simulink model "bench_test_racecar_shiftlight"  (R2023b)
settings: Solver=FixedStepDiscrete  StartTime=0.0  StopTime=inf  FixedStep=0.001  RelTol=1e-3  EnableMultiTasking=on
PreLoadFcn:
  | colow_ws2812
values from neighbouring files (symbols this model uses):
  all_off = [one_off one_off one_off one_off one_off one_off one_off one_off one_off one_off one_off one_off one_off one_off zeros]    [colow_ws2812.m]
  final_drive_ratio = 4.765    [colow_ws2812.m]
  red_day_all = [red_day red_day red_day red_day red_day red_day red_day red_day red_day red_day red_day red_day red_day red_day zeros]    [colow_ws2812.m]
  red_night_all = [red_night red_night red_night red_night red_night red_night red_night red_night red_night red_night red_night red_night red_night red_night zeros]    [colow_ws2812.m]
  stage1_day = [green_day linspace(20,20,288) green_day zeros]    [colow_ws2812.m]
  stage1_night = [green_night linspace(20,20,288) green_night zeros]    [colow_ws2812.m]
  stage2_day = [green_day green_day linspace(20,20,240) green_day green_day zeros]    [colow_ws2812.m]
  stage2_night = [green_night green_night linspace(20,20,240) green_night green_night zeros]    [colow_ws2812.m]
  stage3_day = [green_day green_day red_day linspace(20,20,192) red_day green_day green_day zeros]    [colow_ws2812.m]
  stage3_night = [green_night green_night red_night linspace(20,20,192) red_night green_night green_night zeros]    [colow_ws2812.m]
  stage4_day = [green_day green_day red_day red_day linspace(20,20,144) red_day red_day green_day green_day zeros]    [colow_ws2812.m]
  stage4_night = [green_night green_night red_night red_night linspace(20,20,144) red_night red_night green_night green_night zeros]    [colow_ws2812.m]
  stage5_day = [green_day green_day red_day red_day blue_day linspace(20,20,96) blue_day red_day red_day green_day green_day zeros]    [colow_ws2812.m]
  stage5_night = [green_night green_night red_night red_night blue_night linspace(20,20,96) blue_night red_night red_night green_night green_night zeros]    [colow_ws2812.m]
  stage6_day = [green_day green_day red_day red_day blue_day blue_day linspace(20,20,48) blue_day blue_day red_day red_day green_day green_day zeros]    [colow_ws2812.m]
  stage6_night = [green_night green_night red_night red_night blue_night blue_night linspace(20,20,48) blue_night blue_night red_night red_night green_night green_night zeros]    [colow_ws2812.m]
  stage7_day = [green_day green_day red_day red_day blue_day blue_day blue_day blue_day blue_day blue_day red_day red_day green_day green_day zeros]    [colow_ws2812.m]
  stage7_night = [green_night green_night red_night red_night blue_night blue_night blue_night blue_night blue_night blue_night red_night red_night green_night green_night zeros]    [colow_ws2812.m]
  tire_radius = 0.31265    [colow_ws2812.m]
undefined symbols (not defined in the file or in its folder): Down, epwmFrequency, GPTRIP1SEL, GPTRIP2SEL, TZ1, TZ2, Up
libraries: simulink x18, c2837xDlib x7, c280xlib x4, canmsglib x4, c2802xlib x1
settings Model: ExtModeTrigDuration=8  Creator=LinF  LastModifiedBy=LinF
settings OptimizationCC: DefaultUnderspecifiedDataType=single  EnhancedBackFolding=on  PassReuseOutputArgsAs=Individual arguments  MaxStackSize=1024  OptimizeBlockOrder=speed  DifferentSizesBufferReuse=on  OptimizationCustomize=off  EfficientTunableParamExpr=on
settings DebuggingCC: ParameterTunabilityLossMsg=error
settings HardwareCC: ProdBitPerChar=16  ProdBitPerInt=16  ProdBitPerPointer=32  ProdBitPerSizeT=32  ProdBitPerPtrDiffT=32  ProdLargestAtomicInteger=Integer  ProdLargestAtomicFloat=None  ProdWordSize=16  ProdLongLongMode=on  ProdHWDeviceType=Texas Instruments->C2000  HardwareBoardFeatureSet=SoCBlockset
settings ModelReferenceCC: ModelReferenceNumInstancesAllowed=Single
settings SFSimCC: MATLABDynamicMemAlloc=off
settings RTWCC: Description=Embedded Coder  SystemTargetFile=ert.tlc  HardwareBoard=TI Delfino F28379D LaunchPad  TemplateMakefile=ert_default_tmf  Toolchain=Texas Instruments Code Composer Studio (C2000)  CodeProfilingSaveOptions=MetricsOnly
settings CodeAppCC: ForceParamTrailComments=on  IgnoreCustomStorageClasses=off  OperatorAnnotations=on  SimulinkDataObjDesc=on  SFDataObjDesc=on  InsertBlockDesc=on
settings ERTTargetCC: CodeReplacementLibrary=TI C28x  ExtModeTransport=4  ExtModeStaticAlloc=on  ExtModeAutomaticAllocSize=off  ExtModeStaticAllocSize=10000  ExtModeMexFile=ext_xcp  ExtModeIntrfLevel=Level2 - Open

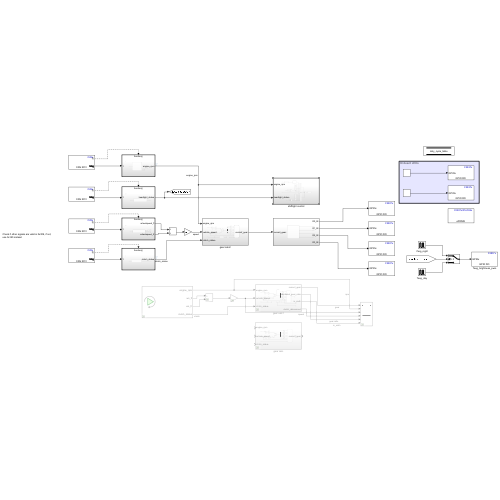
[thumbnail: Simulink's stored preview of the top-level diagram]
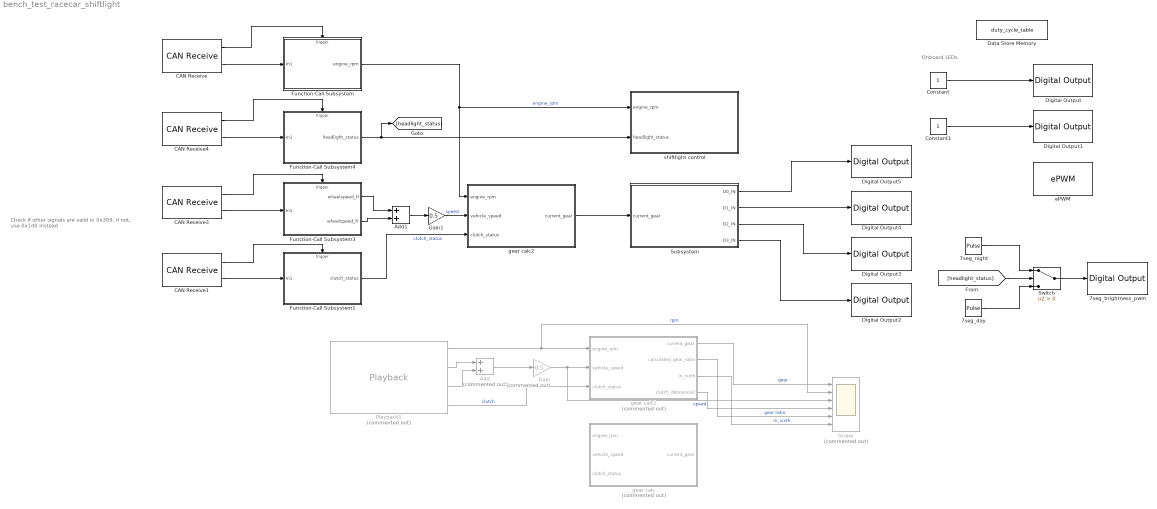
== system bench_test_racecar_shiftlight ==
  note: Check if other signals are valid in 0x309, if not,
      | use 0x1d0 instead
  note: Onboard LEDs
  7seg_brightness_pwm : c2837xDlib/Digital Output  GPIO_Number=GPIO128~GPIO135  GPIO_Bit0=off  GPIO_BIT0_Toggle=off  GPIO_Bit1=off  GPIO_BIT1_Toggle=off  GPIO_Bit2=on  GPIO_BIT2_Toggle=off  GPIO_Bit3=off  GPIO_BIT3_Toggle=off  GPIO_Bit4=off  GPIO_BIT4_Toggle=off  GPIO_Bit5=off  GPIO_BIT5_Toggle=off  GPIO_Bit6=off  GPIO_BIT6_Toggle=off  GPIO_Bit7=off  GPIO_BIT7_Toggle=off
  7seg_day : DiscretePulseGenerator  PulseType=Time based  Period=0.01  PulseWidth=40
  7seg_night : DiscretePulseGenerator  PulseType=Time based  Period=0.01  PulseWidth=90
  Add : Sum  Commented=on
  Add1 : Sum
  CAN Receive : c280xlib/CAN Receive  chipFamily=C280x  useModule=CAN_B  mailboxNo=0  messageID=hex2dec('17c')  messageType=Standard (11-bit identifier)  enableAcceptanceFiltering=off  messageIDMask=0  sampleTime=-1  dataType=CAN_MESSAGE_TYPE  outputAction=Output last received values  initValue=0  outputMessageID=off  outputMessageLength=off  outputMessageTimeStamp=off  postInterrupt=off  interruptLine=0
      settings: LibrarySourceBlock=c2837xDlib/CAN Receive
  CAN Receive1 : c280xlib/CAN Receive  chipFamily=C280x  useModule=CAN_B  mailboxNo=2  messageID=hex2dec('13c')  messageType=Standard (11-bit identifier)  enableAcceptanceFiltering=off  messageIDMask=0  sampleTime=-1  dataType=CAN_MESSAGE_TYPE  outputAction=Output last received values  initValue=0  outputMessageID=off  outputMessageLength=off  outputMessageTimeStamp=off  postInterrupt=off  interruptLine=0
      settings: LibrarySourceBlock=c2837xDlib/CAN Receive
  CAN Receive3 : c280xlib/CAN Receive  chipFamily=C280x  useModule=CAN_B  mailboxNo=3  messageID=hex2dec('1d0')  messageType=Standard (11-bit identifier)  enableAcceptanceFiltering=off  messageIDMask=0  sampleTime=-1  dataType=CAN_MESSAGE_TYPE  outputAction=Output last received values  initValue=0  outputMessageID=off  outputMessageLength=off  outputMessageTimeStamp=off  postInterrupt=off  interruptLine=0
      settings: LibrarySourceBlock=c2837xDlib/CAN Receive
  CAN Receive4 : c280xlib/CAN Receive  chipFamily=C280x  useModule=CAN_B  mailboxNo=4  messageID=hex2dec('164')  messageType=Standard (11-bit identifier)  enableAcceptanceFiltering=off  messageIDMask=0  sampleTime=-1  dataType=CAN_MESSAGE_TYPE  outputAction=Output last received values  initValue=0  outputMessageID=off  outputMessageLength=off  outputMessageTimeStamp=off  postInterrupt=off  interruptLine=0
      settings: LibrarySourceBlock=c2837xDlib/CAN Receive
  Constant : Constant
  Constant1 : Constant
  Data Store Memory : DataStoreMemory  DataStoreName=duty_cycle_table  WriteAfterWriteMsg=warning  InitialValue=all_off  ShowAdditionalParam=off  OutDataTypeStr=uint16  Dimensions=396
  Digital Output : c2837xDlib/Digital Output  GPIO_Number=GPIO24~GPIO31  GPIO_Bit0=off  GPIO_BIT0_Toggle=off  GPIO_Bit1=off  GPIO_BIT1_Toggle=off  GPIO_Bit2=off  GPIO_BIT2_Toggle=off  GPIO_Bit3=off  GPIO_BIT3_Toggle=off  GPIO_Bit4=off  GPIO_BIT4_Toggle=off  GPIO_Bit5=off  GPIO_BIT5_Toggle=off  GPIO_Bit6=off  GPIO_BIT6_Toggle=off  GPIO_Bit7=on  GPIO_BIT7_Toggle=off
  Digital Output1 : c2837xDlib/Digital Output  GPIO_Number=GPIO32~GPIO39  GPIO_Bit0=off  GPIO_BIT0_Toggle=off  GPIO_Bit1=off  GPIO_BIT1_Toggle=off  GPIO_Bit2=on  GPIO_BIT2_Toggle=off  GPIO_Bit3=off  GPIO_BIT3_Toggle=off  GPIO_Bit4=off  GPIO_BIT4_Toggle=off  GPIO_Bit5=off  GPIO_BIT5_Toggle=off  GPIO_Bit6=off  GPIO_BIT6_Toggle=off  GPIO_Bit7=off  GPIO_BIT7_Toggle=off
  Digital Output2 : c2837xDlib/Digital Output  GPIO_Number=GPIO56~GPIO63  GPIO_Bit0=off  GPIO_BIT0_Toggle=off  GPIO_Bit1=off  GPIO_BIT1_Toggle=off  GPIO_Bit2=on  GPIO_BIT2_Toggle=off  GPIO_Bit3=off  GPIO_BIT3_Toggle=off  GPIO_Bit4=off  GPIO_BIT4_Toggle=off  GPIO_Bit5=off  GPIO_BIT5_Toggle=off  GPIO_Bit6=off  GPIO_BIT6_Toggle=off  GPIO_Bit7=off  GPIO_BIT7_Toggle=off
  Digital Output3 : c2837xDlib/Digital Output  GPIO_Number=GPIO56~GPIO63  GPIO_Bit0=off  GPIO_BIT0_Toggle=off  GPIO_Bit1=off  GPIO_BIT1_Toggle=off  GPIO_Bit2=off  GPIO_BIT2_Toggle=off  GPIO_Bit3=on  GPIO_BIT3_Toggle=off  GPIO_Bit4=off  GPIO_BIT4_Toggle=off  GPIO_Bit5=off  GPIO_BIT5_Toggle=off  GPIO_Bit6=off  GPIO_BIT6_Toggle=off  GPIO_Bit7=off  GPIO_BIT7_Toggle=off
  Digital Output4 : c2837xDlib/Digital Output  GPIO_Number=GPIO120~GPIO127  GPIO_Bit0=off  GPIO_BIT0_Toggle=off  GPIO_Bit1=off  GPIO_BIT1_Toggle=off  GPIO_Bit2=off  GPIO_BIT2_Toggle=off  GPIO_Bit3=off  GPIO_BIT3_Toggle=off  GPIO_Bit4=on  GPIO_BIT4_Toggle=off  GPIO_Bit5=off  GPIO_BIT5_Toggle=off  GPIO_Bit6=off  GPIO_BIT6_Toggle=off  GPIO_Bit7=off  GPIO_BIT7_Toggle=off
  Digital Output5 : c2837xDlib/Digital Output  GPIO_Number=GPIO120~GPIO127  GPIO_Bit0=off  GPIO_BIT0_Toggle=off  GPIO_Bit1=off  GPIO_BIT1_Toggle=off  GPIO_Bit2=off  GPIO_BIT2_Toggle=off  GPIO_Bit3=off  GPIO_BIT3_Toggle=off  GPIO_Bit4=off  GPIO_BIT4_Toggle=off  GPIO_Bit5=on  GPIO_BIT5_Toggle=off  GPIO_Bit6=off  GPIO_BIT6_Toggle=off  GPIO_Bit7=off  GPIO_BIT7_Toggle=off
  Function-Call Subsystem : Subsystem  TreatAsAtomicUnit=on
  Function-Call Subsystem1 : Subsystem  TreatAsAtomicUnit=on
  Function-Call Subsystem3 : Subsystem  TreatAsAtomicUnit=on
  Function-Call Subsystem4 : Subsystem  TreatAsAtomicUnit=on
  Gain : Gain  Commented=on  Gain=0.5
  Gain1 : Gain  Gain=0.5
  Playback1 : Playback  Commented=on  NumPorts=4  PartName=793a99b5-5b81-49ab-9d78-3a6aebb216a4
  Scope : Scope  Commented=on  NumInputPorts=6
  Subsystem : Subsystem
  Switch : Switch  Criteria=u2 > Threshold  SaturateOnIntegerOverflow=off  InputSameDT=off
  ePWM : c2802xlib/ePWM  PwmType=C2000_Type4  useModule=ePWM8  ePWMxLINKTBPRD=Not Linked  periodUnits=Clock cycles  timerSource=Specify via dialog  timerPeriod_clk=63  timerPeriod_sec=1/epwmFrequency  tbshadow=Counter equals to zero  countingMode=Up-Down  phaseActiveEnable=Disable  phaseDirection=Count down after sync  phaseActive=0  synchronizationEnable=off  dcaevt1Sync=off  dcbevt1Sync=off  synchronizationOption=Disable  dcbevt1SyncOut=off  dcaevt1SyncOut=off  cmpdSyncOut=off  cmpcSyncOut=off  cmpbSyncOut=off  zeroSyncOut=off  swfSyncOut=off  perSynchronizationOption=Counter equals to period (CTR=PRD)  clockPrescale=1  HSclockPrescale=1  enswap=off  ePWMxAStatus=off  ePWMxAactionLogic1=Set  ePWMxAactionLogic2=Clear  ePWMxAactionLogic3=Clear  ePWMxAactionLogic4=Set  ePWMxAactionLogic5=Do nothing  ePWMxAactionLogic6=Do nothing  ePWMxACSFenable=off  ePWMxACSFvalue=Forcing disable  ePWMxASFreload=Zero  ePWMxBStatus=on  ePWMxBactionLogic1=Set  ePWMxBactionLogic2=Clear  ePWMxBactionLogic3=Clear  ePWMxBactionLogic4=Set  ePWMxBactionLogic5=Do nothing  ePWMxBactionLogic6=Do nothing  ePWMxBCSFenable=off  ePWMxBCSFvalue=Forcing disable  ePWMxBSFreload=Zero  ePWNxBOutWay=off  ePWMxLINKCMPA=ePWM8  CMPAUnits=Percentages  CMPASource=Specify via dialog  CMPAValue_per=50  CMPAValue_clk=32000  enCMPAshadow=Counter equals to zero (CTR=Zero)  ePWMxLINKCMPB=Not Linked  CMPBUnits=Clock cycles  CMPBSource=Specify via dialog  CMPBValue_per=50  CMPBValue_clk=32000  enCMPBshadow=Counter equals to zero (CTR=Zero)  ePWMxLINKCMPC=Not Linked  CMPCUnits=Clock cycles  CMPCSource=Specify via dialog  CMPCValue_per=50  CMPCValue_clk=32000  enCMPCshadow=Counter equals to zero (CTR=Zero)  ePWMxLINKCMPD=Not Linked  CMPDUnits=Clock cycles  CMPDSource=Specify via dialog  CMPDValue_per=50  CMPDValue_clk=32000  enCMPDshadow=Counter equals to zero (CTR=Zero)  enableDBePWMxA=off  enableDBePWMxB=off  enhalfcycle=off  DBpolarity=Active high (AH)  DBedgeDelay=Positive  DBSource_ePWMxA=ePWMxA  DBSource_ePWMxB=ePWMxA  DBPeriodUnits=Clock cycles  DBperiodSource=Specify via dialog  REDperiod=0  FEDperiod=0  REDperiod_sec=0  FEDperiod_sec=0  LoadModeDBRED=Immediate without using shadow  LoadModeDBFED=Immediate without using shadow  adcstartModuleA=on  adcrequestEventA=First event  adcstartEventA=Digital Compare Module A Event 1 start of conversion (DCAEVT1.soc)  adcstartEventA_type2=Counter equals to period (CTR=PRD)  adcstartModuleB=off  adcrequestEventB=First event  adcstartEventB=Counter equals to zero (CTR=Zero)  adcstartEventB_type2=Counter equals to zero (CTR=Zero)  intEn=off  intPrd=First event  intSel=Counter equals to zero (CTR=Zero)  intSel_type2=Counter equals to zero (CTR=Zero)  hrpe=off  enHRPWM=off  HRPWM_LoadMode=Counter equals to period (CTR=PRD)  HRPWM_CTLMode=Duty or Period control mode  HRPWM_EDGMode=Both edge  hrpeb=off  enHRPWMB=off  HRPWM_LoadModeB=Counter equals to zero (CTR=ZERO)  HRPWM_CTLModeB=Duty or Period control mode  HRPWM_EDGModeB=Both edge  enHRDBRED=off  enHRDBFED=off  enSFO=on  enautoconv=on  chopperEnable=off  chopperFrequency=1  chopperFirstwidth=1  chopperDuty=12.5%  tripZonesource=Specify via dialog  tzselOSHT1=off  tzselOSHT2=off  tzselOSHT3=off  tzselOSHDCAEV1=off  tzselOSHDCBEV1=off  tzselCBC1=off  tzselCBC2=off  tzselCBC3=off  tzselCBCDCAEV2=off  tzselCBCDCBEV2=off  tzselOSHT4=off  tzselOSHT5=off  tzselOSHT6=off  tzselCBC4=off  tzselCBC5=off  tzselCBC6=off  enTzOstIntr=off  enTzCbcIntr=off  enTzDCAEVT1Intr=off  enTzDCAEVT2Intr=off  enTzDCBEVT1Intr=off  enTzDCBEVT2Intr=off  ePWMxAforced=No action  ePWMxBforced=No action  DCAEVT1forced=No action  DCBEVT1forced=No action  DCAEVT2forced=No action  DCBEVT2forced=No action  dcah=Trip Zone 1 input (TZ1)  dcal=Trip Zone 2 input (TZ2)  dcbh=Trip Zone 1 input (TZ1)  dcbl=Trip Zone 2 input (TZ2)  dcah_type2=GPTRIP1SEL/(TZ1)  dcal_type2=GPTRIP2SEL/(TZ2)  dcbh_type2=GPTRIP1SEL/(TZ1)  dcbl_type2=GPTRIP2SEL/(TZ2)  gendcaevt1=Event disabled  gendcaevt2=Event disabled  gendcbevt1=Event disabled  gendcbevt2=Event disabled  dcaevt1src=DCAEVT1 with sync  dcaevt2src=DCAEVT2 with sync  dcbevt1src=DCBEVT1 with sync  dcbevt2src=DCBEVT2 with sync  pulsesel=Counter equals to zero (CTR=Zero)  blankinv=off  blankoffset=0  blankwidth=0  evsrcsel=Filtered version of DCAEVT1 (DCAEVT1FILT)  encape=off
  gear calc : Subsystem  Commented=on
  gear calc1 : Subsystem  Commented=on
  gear calc2 : Subsystem
  shiftlight control : Subsystem
  wires:
  Constant/1 -> Digital Output/1
  Constant1/1 -> Digital Output1/1
  CAN Receive/2 -> Function-Call Subsystem/1(In1)
  CAN Receive/1 -> Function-Call Subsystem/Trigger
  Function-Call Subsystem/1(engine_rpm) -> gear calc2/1(engine_rpm), shiftlight control/1(engine_rpm)  "engine_rpm"
  CAN Receive1/2 -> Function-Call Subsystem1/1(In1)
  CAN Receive1/1 -> Function-Call Subsystem1/Trigger
  Function-Call Subsystem1/1(clutch_status) -> gear calc2/3(clutch_status)  "clutch_status"
  CAN Receive3/2 -> Function-Call Subsystem3/1(In1)
  CAN Receive3/1 -> Function-Call Subsystem3/Trigger
  CAN Receive4/1 -> Function-Call Subsystem4/Trigger
  CAN Receive4/2 -> Function-Call Subsystem4/1(In1)
  Playback1/1 -> Scope/2, gear calc1/1(engine_rpm)  "rpm"
  Playback1/2 -> Add/1
  Playback1/3 -> Add/2
  Add/1 -> Gain/1
  Gain/1 -> Scope/3, gear calc1/2(vehicle_speed)  "speed"
  Playback1/4 -> gear calc1/3(clutch_status)  "clutch"
  gear calc1/1(current_gear) -> Scope/1  "gear"
  gear calc1/2(calculated_gear_ratio) -> Scope/5  "gear ratio"
  gear calc1/3(in_sixth) -> Scope/6  "in_sixth"
  gear calc1/4(clutch_debounced) -> Scope/4
  Add1/1 -> Gain1/1
  Gain1/1 -> gear calc2/2(vehicle_speed)  "speed"
  Function-Call Subsystem3/1(wheelspeed_fl) -> Add1/1
  Function-Call Subsystem3/2(wheelspeed_fr) -> Add1/2
  Subsystem/4(D3_IN) -> Digital Output2/1
  Subsystem/3(D2_IN) -> Digital Output3/1
  Subsystem/2(D1_IN) -> Digital Output4/1
  Subsystem/1(D0_IN) -> Digital Output5/1
  gear calc2/1(current_gear) -> Subsystem/1(current_gear)
  Switch/1 -> 7seg_brightness_pwm/1
  [headlight_status] -> Switch/2
  7seg_night/1 -> Switch/1
  7seg_day/1 -> Switch/3
  Function-Call Subsystem4/1(headlight_status) -> shiftlight control/2(headlight_status), [headlight_status]

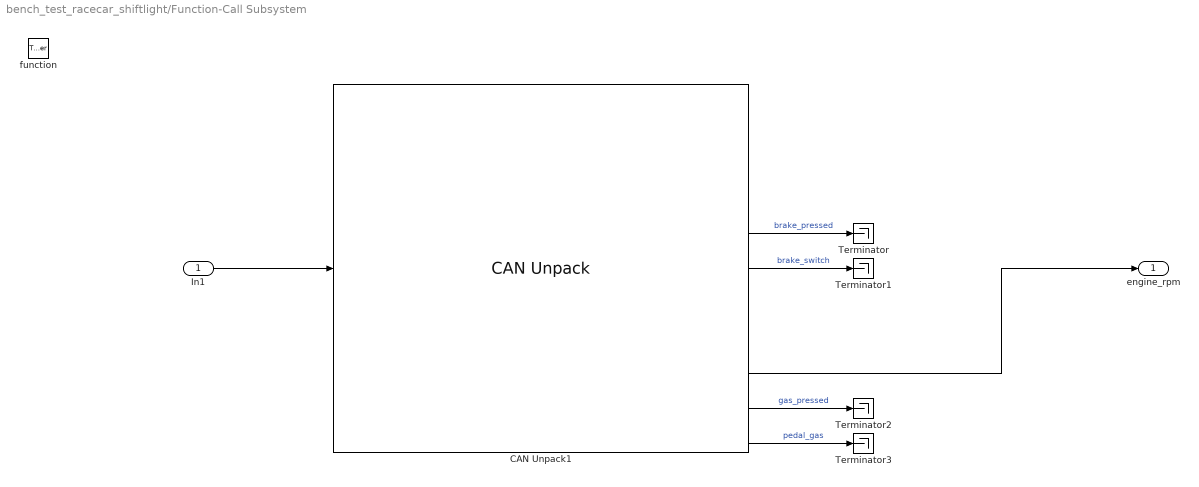
== system bench_test_racecar_shiftlight/Function-Call Subsystem ==
  In1 : Inport
  function : TriggerPort  TriggerType=function-call  VariantControl=(inherit)
  CAN Unpack1 : canmsglib/CAN Unpack  CANdbFile=C:\school\racecar_shiftlight\acura_ilx_2013.dbc  MsgList=POWERTRAIN_DATA  MsgName=POWERTRAIN_DATA  MsgIDType=Standard (11-bit identifier)  MsgIdentifier=380  MsgLength=8  SignalInfo={'ACC_STATUS','38','1','BE','unsigned','Standard','0','1','0','0','1';'BOH2_17C','54','10','BE','unsigned','Standard','0','1','0','0','1';'BOH3_17C','48','5','BE','unsigned','Standard','0','1','0','0','1';'BOH_17C','33','5','BE','unsigned','Standard','0','1','0','0','1';'BRAKE_PRESSED','53','1','BE','unsigned','Standard','0','1','0','0','1';'BRAKE_SWITCH','32','1','BE','unsigned','Standard','0','1','0','0','1';'CHECKSUM','56','4','BE','unsigned','Standard','0','1','0','0','15';'COUNTER','60','2','BE','unsigned','Standard','0','1','0','0','3';'ENGINE_RPM','24','16','BE','unsigned','Standard','0','1','0','0','65535';'GAS_PRESSED','39','1','BE','unsigned','Standard','0','1','0','0','1';'PEDAL_GAS','0','8','BE','unsigned','Standard','0','1','0','0','255'}  IDPort=off  TimestampPort=off  ErrorPort=off  RemotePort=off  LengthPort=off  StatusPort=off  ApplyMinMax=off
      settings: LibrarySourceBlock=c2000lib/Target Communication/CAN Unpack  DataFormat=CANdb specified signals
  Terminator{,1..3} (4 alike) : Terminator
  engine_rpm : Outport
  wires:
  In1/1 -> CAN Unpack1/1
  CAN Unpack1/5 -> Terminator/1  "brake_pressed"
  CAN Unpack1/6 -> Terminator1/1  "brake_switch"
  CAN Unpack1/9 -> engine_rpm/1
  CAN Unpack1/10 -> Terminator2/1  "gas_pressed"
  CAN Unpack1/11 -> Terminator3/1  "pedal_gas"

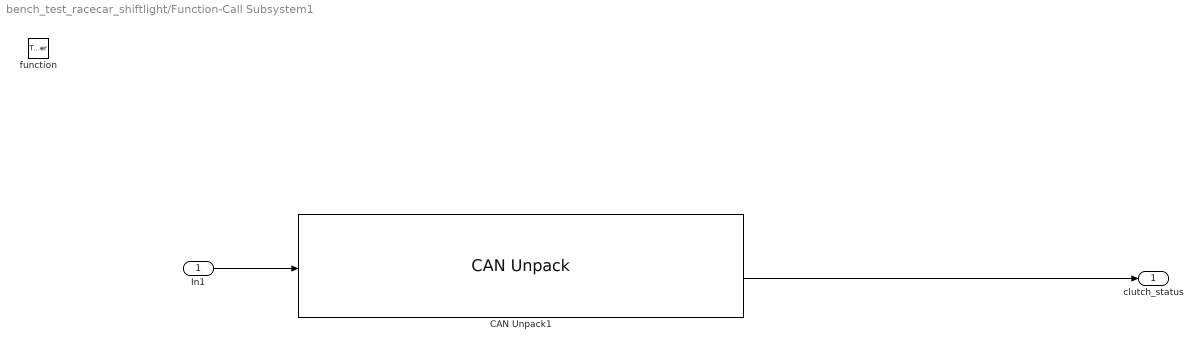
== system bench_test_racecar_shiftlight/Function-Call Subsystem1 ==
  In1 : Inport
  function : TriggerPort  TriggerType=function-call  VariantControl=(inherit)
  CAN Unpack1 : canmsglib/CAN Unpack  CANdbFile=C:\school\racecar_shiftlight\acura_ilx_2013.dbc  MsgList=GAS_PEDAL  MsgName=GAS_PEDAL  MsgIDType=Standard (11-bit identifier)  MsgIdentifier=316  MsgLength=8  SignalInfo={'CAR_GAS','32','8','BE','unsigned','Standard','0','1','0','0','255';'CHECKSUM','56','4','BE','unsigned','Standard','0','1','0','0','15';'CLUTCH_STATUS_n','50','1','BE','unsigned','Standard','0','1','0','0','1';'COUNTER','60','2','BE','unsigned','Standard','0','1','0','0','3'}  IDPort=off  TimestampPort=off  ErrorPort=off  RemotePort=off  LengthPort=off  StatusPort=off  ApplyMinMax=off
      settings: LibrarySourceBlock=c2000lib/Target Communication/CAN Unpack  DataFormat=CANdb specified signals
  clutch_status : Outport
  wires:
  In1/1 -> CAN Unpack1/1
  CAN Unpack1/3 -> clutch_status/1

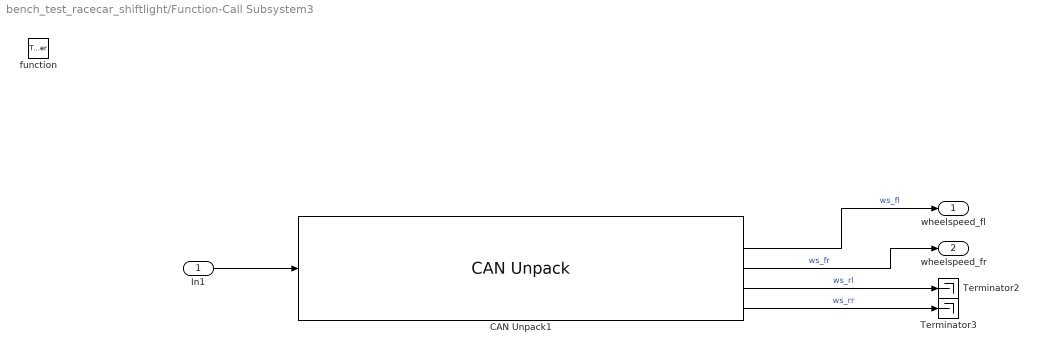
== system bench_test_racecar_shiftlight/Function-Call Subsystem3 ==
  In1 : Inport
  function : TriggerPort  TriggerType=function-call  VariantControl=(inherit)
  CAN Unpack1 : canmsglib/CAN Unpack  CANdbFile=C:\school\racecar_shiftlight\acura_ilx_2013.dbc  MsgList=WHEEL_SPEEDS  MsgName=WHEEL_SPEEDS  MsgIDType=Standard (11-bit identifier)  MsgIdentifier=464  MsgLength=8  SignalInfo={'CHECKSUM','56','4','BE','unsigned','Standard','0','1','0','0','3';'WHEEL_SPEED_FL','9','15','BE','unsigned','Standard','0','0.01','0','0','250';'WHEEL_SPEED_FR','26','15','BE','unsigned','Standard','0','0.01','0','0','250';'WHEEL_SPEED_RL','43','15','BE','unsigned','Standard','0','0.01','0','0','250';'WHEEL_SPEED_RR','60','15','BE','unsigned','Standard','0','0.01','0','0','250'}  IDPort=off  TimestampPort=off  ErrorPort=off  RemotePort=off  LengthPort=off  StatusPort=off  ApplyMinMax=off
      settings: LibrarySourceBlock=c2000lib/Target Communication/CAN Unpack  DataFormat=CANdb specified signals
  Terminator2 : Terminator
  Terminator3 : Terminator
  wheelspeed_fl : Outport
  wheelspeed_fr : Outport  Port=2
  wires:
  In1/1 -> CAN Unpack1/1
  CAN Unpack1/2 -> wheelspeed_fl/1  "ws_fl"
  CAN Unpack1/3 -> wheelspeed_fr/1  "ws_fr"
  CAN Unpack1/4 -> Terminator2/1  "ws_rl"
  CAN Unpack1/5 -> Terminator3/1  "ws_rr"

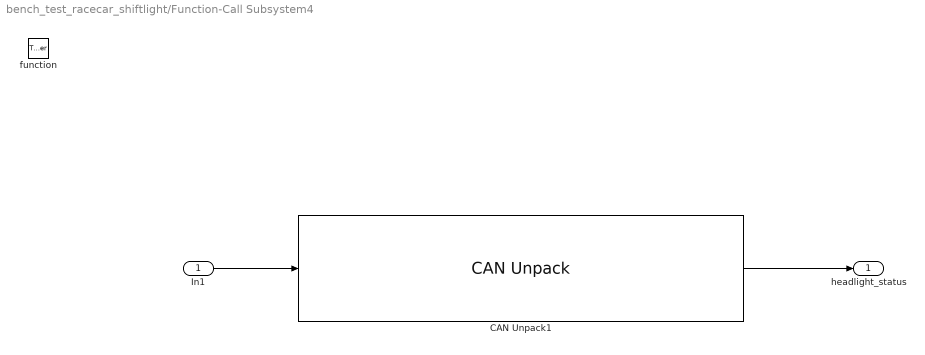
== system bench_test_racecar_shiftlight/Function-Call Subsystem4 ==
  In1 : Inport
  function : TriggerPort  TriggerType=function-call  VariantControl=(inherit)
  CAN Unpack1 : canmsglib/CAN Unpack  CANdbFile=C:\school\racecar_shiftlight\acura_ilx_2013.dbc  MsgList=HEADLIGHT_STATUS  MsgName=HEADLIGHT_STATUS  MsgIDType=Standard (11-bit identifier)  MsgIdentifier=356  MsgLength=8  SignalInfo={'LOW_BEAM_STATUS','1','1','LE','unsigned','Standard','0','1','0','0','1'}  IDPort=off  TimestampPort=off  ErrorPort=off  RemotePort=off  LengthPort=off  StatusPort=off  ApplyMinMax=off
      settings: LibrarySourceBlock=c2000lib/Target Communication/CAN Unpack  DataFormat=CANdb specified signals
  headlight_status : Outport
  wires:
  In1/1 -> CAN Unpack1/1
  CAN Unpack1/1 -> headlight_status/1

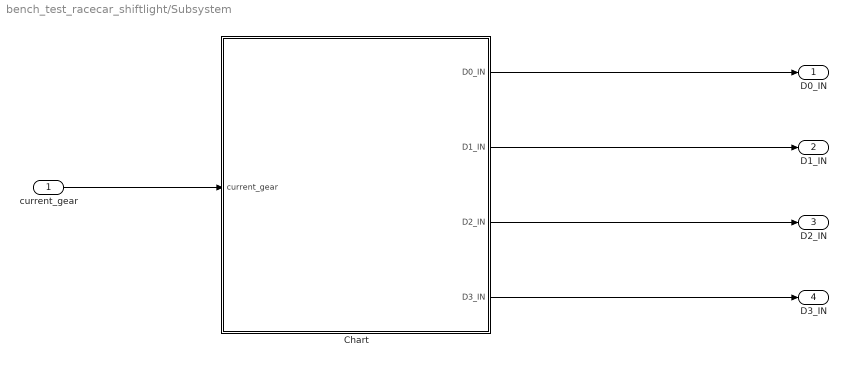
== system bench_test_racecar_shiftlight/Subsystem ==
  current_gear : Inport
  Chart : Stateflow chart  TreatAsAtomicUnit=on
  D0_IN : Outport
  D1_IN : Outport  Port=2
  D2_IN : Outport  Port=3
  D3_IN : Outport  Port=4
  wires:
  current_gear/1 -> Chart/1(current_gear)
  Chart/1(D0_IN) -> D0_IN/1
  Chart/2(D1_IN) -> D1_IN/1
  Chart/3(D2_IN) -> D2_IN/1
  Chart/4(D3_IN) -> D3_IN/1

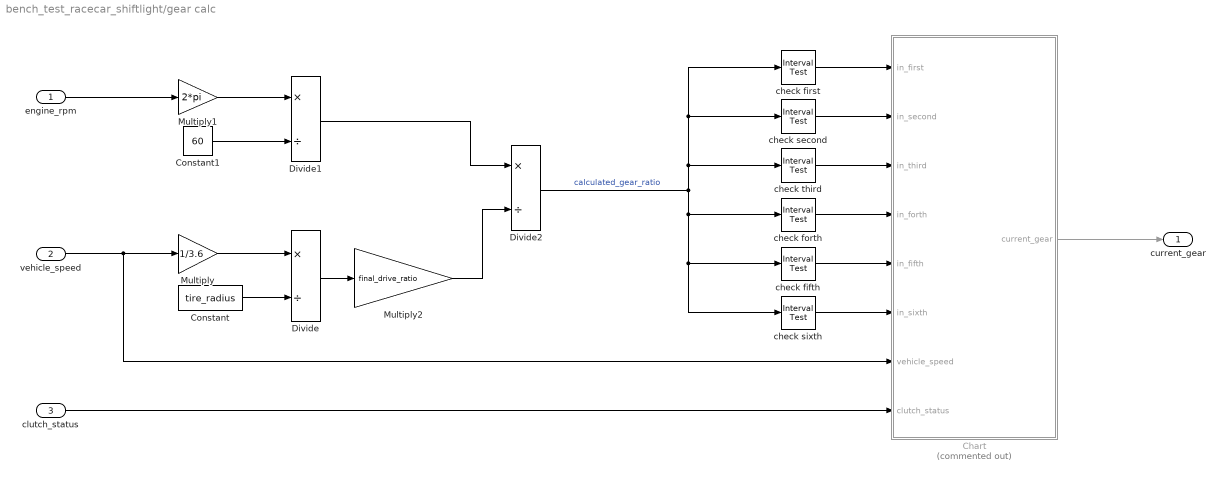
== system bench_test_racecar_shiftlight/gear calc ==
  engine_rpm : Inport
  vehicle_speed : Inport  Port=2
  clutch_status : Inport  Port=3
  Chart : Stateflow chart  Commented=on  TreatAsAtomicUnit=on
      settings: PortSchema="{\"entries\":[{\"content\":{\"sides\":[{\"content\":{\"connectorIds\":[\"In2\",\"In1\",\"In3\",\"In4\",\"In5\",\"In6\",\"In7\",\"In8\"]},\"type\":\"ConnectorPlacement.EquallySpacedRectSide\",\"uuid\":\"7c5ecf18-4ca5-48cf-b6cc-f6d674adc791\"},{\"content\":{\"connectorIds\":[\"Out1\"],\"side\":\"RIGHT\"},\"type\":\"ConnectorPlacement.EquallySpacedRectSide\",\"uuid\":\"8bc4c731-54ce-4b60-a017-d200a54467ca\"},{\"content\":{\"side\":\"TOP\"},\"type\":\"ConnectorPlacement.EquallySpacedRectSide\",\"uuid\":\"b495a058-1853-40c7-b3b0-00e858c713fd\"}]},\"type\":\"ConnectorPlacement.EquallySpacedConnector\",\"uuid\":\"e858d52b-2e7f-42dc-8e65-b599dcab11be\"}],\"packageUris\":[\"http://schema.mathworks.com/mf0/Connector/R2020b\"],\"version\":\"1.0\"}"
  Constant : Constant  Value=tire_radius
  Constant1 : Constant  Value=60
  Divide : Product  Inputs=*/
  Divide1 : Product  Inputs=*/
  Divide2 : Product  Inputs=*/
  Multiply : Gain  Gain=1/3.6
  Multiply1 : Gain  Gain=2*pi
  Multiply2 : Gain  Gain=final_drive_ratio
  check fifth : simulink/Logic and Bit Operations/Interval Test  IntervalClosedRight=on  uplimit=10  IntervalClosedLeft=on  lowlimit=0  OutDataTypeStr=boolean
  check first : simulink/Logic and Bit Operations/Interval Test  IntervalClosedRight=on  uplimit=10  IntervalClosedLeft=on  lowlimit=0  OutDataTypeStr=boolean
  check forth : simulink/Logic and Bit Operations/Interval Test  IntervalClosedRight=on  uplimit=10  IntervalClosedLeft=on  lowlimit=0  OutDataTypeStr=boolean
  check second : simulink/Logic and Bit Operations/Interval Test  IntervalClosedRight=on  uplimit=10  IntervalClosedLeft=on  lowlimit=0  OutDataTypeStr=boolean
  check sixth : simulink/Logic and Bit Operations/Interval Test  IntervalClosedRight=on  uplimit=10  IntervalClosedLeft=on  lowlimit=0  OutDataTypeStr=boolean
  check third : simulink/Logic and Bit Operations/Interval Test  IntervalClosedRight=on  uplimit=10  IntervalClosedLeft=on  lowlimit=0  OutDataTypeStr=boolean
  current_gear : Outport
  wires:
  vehicle_speed/1 -> Chart/7(vehicle_speed), Multiply/1
  Multiply/1 -> Divide/1
  Constant/1 -> Divide/2
  Multiply1/1 -> Divide1/1
  Constant1/1 -> Divide1/2
  engine_rpm/1 -> Multiply1/1
  Divide1/1 -> Divide2/1
  Divide2/1 -> check third/1, check first/1, check second/1, check forth/1, check fifth/1, check sixth/1  "calculated_gear_ratio"
  Divide/1 -> Multiply2/1
  Multiply2/1 -> Divide2/2
  check first/1 -> Chart/2(in_first)
  check second/1 -> Chart/1(in_second)
  check third/1 -> Chart/3(in_third)
  check forth/1 -> Chart/4(in_forth)
  check fifth/1 -> Chart/5(in_fifth)
  check sixth/1 -> Chart/6(in_sixth)
  Chart/1(current_gear) -> current_gear/1
  clutch_status/1 -> Chart/8(clutch_status)

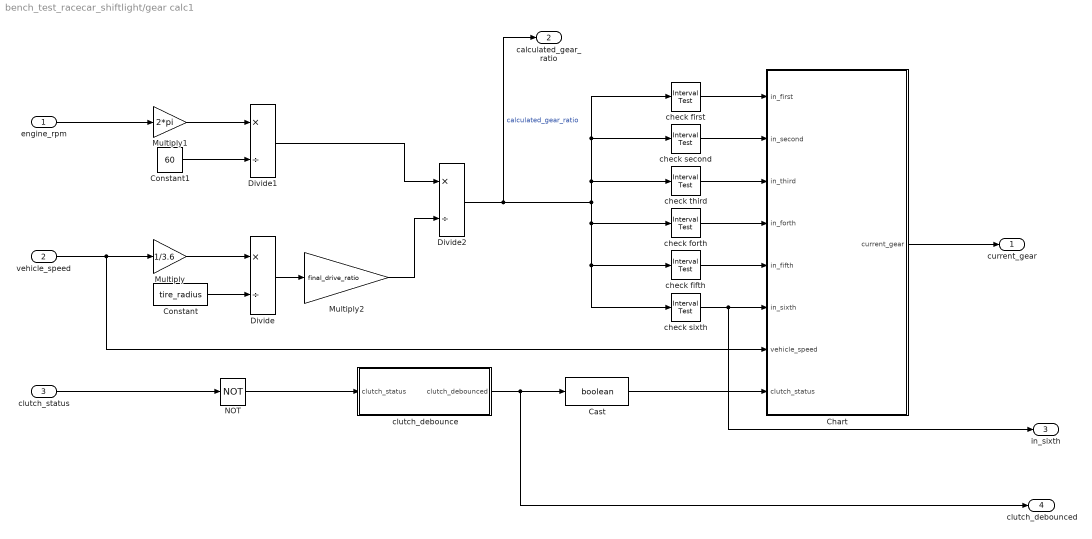
== system bench_test_racecar_shiftlight/gear calc1 ==
  engine_rpm : Inport
  vehicle_speed : Inport  Port=2
  clutch_status : Inport  Port=3
  Cast : DataTypeConversion  OutDataTypeStr=boolean  SaturateOnIntegerOverflow=off  RndMeth=Floor
  Chart : Stateflow chart  TreatAsAtomicUnit=on
      settings: PortSchema="{\"entries\":[{\"content\":{\"sides\":[{\"content\":{\"connectorIds\":[\"In2\",\"In1\",\"In3\",\"In4\",\"In5\",\"In6\",\"In7\",\"In8\"]},\"type\":\"ConnectorPlacement.EquallySpacedRectSide\",\"uuid\":\"7c5ecf18-4ca5-48cf-b6cc-f6d674adc791\"},{\"content\":{\"connectorIds\":[\"Out1\"],\"side\":\"RIGHT\"},\"type\":\"ConnectorPlacement.EquallySpacedRectSide\",\"uuid\":\"8bc4c731-54ce-4b60-a017-d200a54467ca\"},{\"content\":{\"side\":\"TOP\"},\"type\":\"ConnectorPlacement.EquallySpacedRectSide\",\"uuid\":\"b495a058-1853-40c7-b3b0-00e858c713fd\"}]},\"type\":\"ConnectorPlacement.EquallySpacedConnector\",\"uuid\":\"e858d52b-2e7f-42dc-8e65-b599dcab11be\"}],\"packageUris\":[\"http://schema.mathworks.com/mf0/Connector/R2020b\"],\"version\":\"1.0\"}"
  Constant : Constant  Value=tire_radius
  Constant1 : Constant  Value=60
  Divide : Product  Inputs=*/
  Divide1 : Product  Inputs=*/
  Divide2 : Product  Inputs=*/
  Multiply : Gain  Gain=1/3.6
  Multiply1 : Gain  Gain=2*pi
  Multiply2 : Gain  Gain=final_drive_ratio
  NOT : Logic  Operator=NOT  IconShape=distinctive  AllPortsSameDT=off  OutDataTypeStr=boolean
  check fifth : simulink/Logic and Bit Operations/Interval Test  IntervalClosedRight=on  uplimit=0.88  IntervalClosedLeft=on  lowlimit=0.82  OutDataTypeStr=boolean
  check first : simulink/Logic and Bit Operations/Interval Test  IntervalClosedRight=on  uplimit=3.5  IntervalClosedLeft=on  lowlimit=3.1  OutDataTypeStr=boolean
  check forth : simulink/Logic and Bit Operations/Interval Test  IntervalClosedRight=on  uplimit=1.15  IntervalClosedLeft=on  lowlimit=1.05  OutDataTypeStr=boolean
  check second : simulink/Logic and Bit Operations/Interval Test  IntervalClosedRight=on  uplimit=2.19  IntervalClosedLeft=on  lowlimit=1.94  OutDataTypeStr=boolean
  check sixth : simulink/Logic and Bit Operations/Interval Test  IntervalClosedRight=on  uplimit=0.69  IntervalClosedLeft=on  lowlimit=0.63  OutDataTypeStr=boolean
  check third : simulink/Logic and Bit Operations/Interval Test  IntervalClosedRight=on  uplimit=1.55  IntervalClosedLeft=on  lowlimit=1.4  OutDataTypeStr=boolean
  clutch_debounce : Stateflow chart  TreatAsAtomicUnit=on
  current_gear : Outport
  calculated_gear_ratio : Outport  Port=2
  in_sixth : Outport  Port=3
  clutch_debounced : Outport  Port=4
  wires:
  vehicle_speed/1 -> Chart/7(vehicle_speed), Multiply/1
  Multiply/1 -> Divide/1
  Constant/1 -> Divide/2
  Multiply1/1 -> Divide1/1
  Constant1/1 -> Divide1/2
  engine_rpm/1 -> Multiply1/1
  Divide1/1 -> Divide2/1
  Divide2/1 -> calculated_gear_ratio/1, check third/1, check first/1, check second/1, check forth/1, check fifth/1, check sixth/1  "calculated_gear_ratio"
  Divide/1 -> Multiply2/1
  Multiply2/1 -> Divide2/2
  check first/1 -> Chart/2(in_first)
  check second/1 -> Chart/1(in_second)
  check third/1 -> Chart/3(in_third)
  check forth/1 -> Chart/4(in_forth)
  check fifth/1 -> Chart/5(in_fifth)
  check sixth/1 -> in_sixth/1, Chart/6(in_sixth)
  clutch_status/1 -> NOT/1
  clutch_debounce/1(clutch_debounced) -> clutch_debounced/1, Cast/1
  NOT/1 -> clutch_debounce/1(clutch_status)
  Chart/1(current_gear) -> current_gear/1
  Cast/1 -> Chart/8(clutch_status)

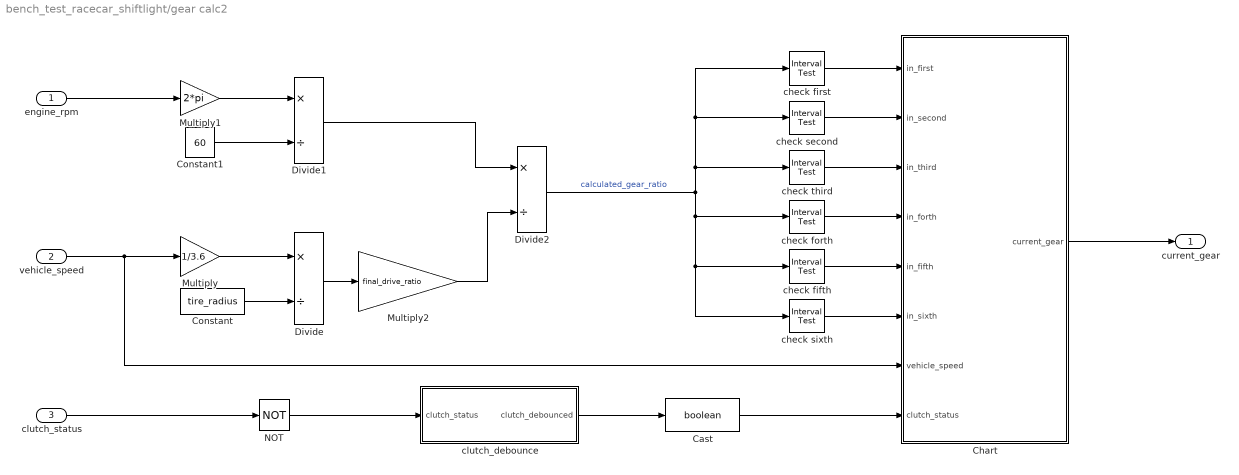
== system bench_test_racecar_shiftlight/gear calc2 ==
  engine_rpm : Inport
  vehicle_speed : Inport  Port=2
  clutch_status : Inport  Port=3
  Cast : DataTypeConversion  OutDataTypeStr=boolean  SaturateOnIntegerOverflow=off  RndMeth=Floor
  Chart : Stateflow chart  TreatAsAtomicUnit=on
      settings: PortSchema="{\"entries\":[{\"content\":{\"sides\":[{\"content\":{\"connectorIds\":[\"In2\",\"In1\",\"In3\",\"In4\",\"In5\",\"In6\",\"In7\",\"In8\"]},\"type\":\"ConnectorPlacement.EquallySpacedRectSide\",\"uuid\":\"7c5ecf18-4ca5-48cf-b6cc-f6d674adc791\"},{\"content\":{\"connectorIds\":[\"Out1\"],\"side\":\"RIGHT\"},\"type\":\"ConnectorPlacement.EquallySpacedRectSide\",\"uuid\":\"8bc4c731-54ce-4b60-a017-d200a54467ca\"},{\"content\":{\"side\":\"TOP\"},\"type\":\"ConnectorPlacement.EquallySpacedRectSide\",\"uuid\":\"b495a058-1853-40c7-b3b0-00e858c713fd\"}]},\"type\":\"ConnectorPlacement.EquallySpacedConnector\",\"uuid\":\"e858d52b-2e7f-42dc-8e65-b599dcab11be\"}],\"packageUris\":[\"http://schema.mathworks.com/mf0/Connector/R2020b\"],\"version\":\"1.0\"}"
  Constant : Constant  Value=tire_radius
  Constant1 : Constant  Value=60
  Divide : Product  Inputs=*/
  Divide1 : Product  Inputs=*/
  Divide2 : Product  Inputs=*/
  Multiply : Gain  Gain=1/3.6
  Multiply1 : Gain  Gain=2*pi
  Multiply2 : Gain  Gain=final_drive_ratio
  NOT : Logic  Operator=NOT  IconShape=distinctive  AllPortsSameDT=off  OutDataTypeStr=boolean
  check fifth : simulink/Logic and Bit Operations/Interval Test  IntervalClosedRight=on  uplimit=0.88  IntervalClosedLeft=on  lowlimit=0.82  OutDataTypeStr=boolean
  check first : simulink/Logic and Bit Operations/Interval Test  IntervalClosedRight=on  uplimit=3.5  IntervalClosedLeft=on  lowlimit=3.1  OutDataTypeStr=boolean
  check forth : simulink/Logic and Bit Operations/Interval Test  IntervalClosedRight=on  uplimit=1.15  IntervalClosedLeft=on  lowlimit=1.05  OutDataTypeStr=boolean
  check second : simulink/Logic and Bit Operations/Interval Test  IntervalClosedRight=on  uplimit=2.19  IntervalClosedLeft=on  lowlimit=1.94  OutDataTypeStr=boolean
  check sixth : simulink/Logic and Bit Operations/Interval Test  IntervalClosedRight=on  uplimit=0.69  IntervalClosedLeft=on  lowlimit=0.63  OutDataTypeStr=boolean
  check third : simulink/Logic and Bit Operations/Interval Test  IntervalClosedRight=on  uplimit=1.55  IntervalClosedLeft=on  lowlimit=1.4  OutDataTypeStr=boolean
  clutch_debounce : Stateflow chart  TreatAsAtomicUnit=on
  current_gear : Outport
  wires:
  Cast/1 -> Chart/8(clutch_status)
  Chart/1(current_gear) -> current_gear/1
  NOT/1 -> clutch_debounce/1(clutch_status)
  clutch_debounce/1(clutch_debounced) -> Cast/1
  clutch_status/1 -> NOT/1
  check sixth/1 -> Chart/6(in_sixth)
  check fifth/1 -> Chart/5(in_fifth)
  check forth/1 -> Chart/4(in_forth)
  check third/1 -> Chart/3(in_third)
  check second/1 -> Chart/1(in_second)
  check first/1 -> Chart/2(in_first)
  Multiply2/1 -> Divide2/2
  Divide/1 -> Multiply2/1
  Divide2/1 -> check sixth/1, check fifth/1, check forth/1, check second/1, check first/1, check third/1  "calculated_gear_ratio"
  Divide1/1 -> Divide2/1
  engine_rpm/1 -> Multiply1/1
  Constant1/1 -> Divide1/2
  Multiply1/1 -> Divide1/1
  Constant/1 -> Divide/2
  Multiply/1 -> Divide/1
  vehicle_speed/1 -> Multiply/1, Chart/7(vehicle_speed)

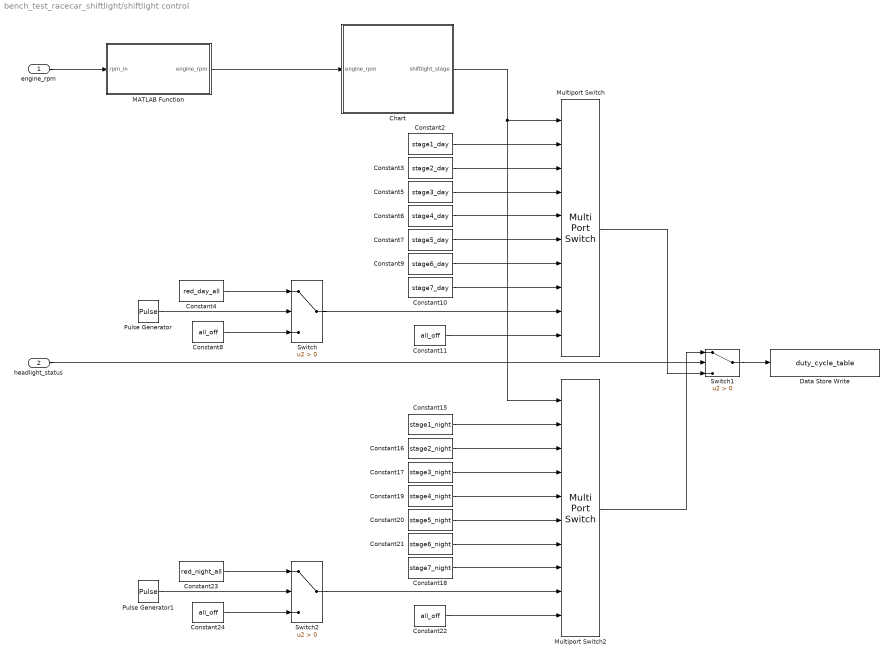
== system bench_test_racecar_shiftlight/shiftlight control ==
  engine_rpm : Inport
  headlight_status : Inport  Port=2
  Chart : Stateflow chart  TreatAsAtomicUnit=on
  Constant10 : Constant  Value=stage7_day  OutDataTypeStr=uint16
  Constant{8,11,22,24} (4 alike) : Constant  Value=all_off  OutDataTypeStr=uint16
  Constant15 : Constant  Value=stage1_night  OutDataTypeStr=uint16
  Constant16 : Constant  Value=stage2_night  OutDataTypeStr=uint16
  Constant17 : Constant  Value=stage3_night  OutDataTypeStr=uint16
  Constant18 : Constant  Value=stage7_night  OutDataTypeStr=uint16
  Constant19 : Constant  Value=stage4_night  OutDataTypeStr=uint16
  Constant2 : Constant  Value=stage1_day  OutDataTypeStr=uint16
  Constant20 : Constant  Value=stage5_night  OutDataTypeStr=uint16
  Constant21 : Constant  Value=stage6_night  OutDataTypeStr=uint16
  Constant23 : Constant  Value=red_night_all  OutDataTypeStr=uint16
  Constant3 : Constant  Value=stage2_day  OutDataTypeStr=uint16
  Constant4 : Constant  Value=red_day_all  OutDataTypeStr=uint16
  Constant5 : Constant  Value=stage3_day  OutDataTypeStr=uint16
  Constant6 : Constant  Value=stage4_day  OutDataTypeStr=uint16
  Constant7 : Constant  Value=stage5_day  OutDataTypeStr=uint16
  Constant9 : Constant  Value=stage6_day  OutDataTypeStr=uint16
  Data Store Write : DataStoreWrite  DataStoreName=duty_cycle_table  IndexOptions=Index vector (dialog)  Indices=1  OutputSizes=1
  MATLAB Function : MATLAB Function  TreatAsAtomicUnit=on
  Multiport Switch : MultiPortSwitch  Inputs=9  DataPortIndices={5500,6000,6500,6800,0}  DiagnosticForDefault=Warning  SaturateOnIntegerOverflow=off  InputSameDT=off
  Multiport Switch2 : MultiPortSwitch  Inputs=9  DataPortIndices={5500,6000,6500,6800,0}  DiagnosticForDefault=Warning  SaturateOnIntegerOverflow=off  InputSameDT=off
  Pulse Generator : DiscretePulseGenerator  PulseType=Time based  Period=0.15  PulseWidth=50
  Pulse Generator1 : DiscretePulseGenerator  PulseType=Time based  Period=0.15  PulseWidth=50
  Switch : Switch  Criteria=u2 > Threshold  SaturateOnIntegerOverflow=off  InputSameDT=off
  Switch1 : Switch  Criteria=u2 > Threshold  SaturateOnIntegerOverflow=off  InputSameDT=off
  Switch2 : Switch  Criteria=u2 > Threshold  SaturateOnIntegerOverflow=off  InputSameDT=off
  wires:
  Pulse Generator/1 -> Switch/2
  Constant9/1 -> Multiport Switch/7
  Constant11/1 -> Multiport Switch/10
  Constant6/1 -> Multiport Switch/5
  Chart/1(shiftlight_stage) -> Multiport Switch2/1, Multiport Switch/1
  Constant10/1 -> Multiport Switch/8
  Constant8/1 -> Switch/3
  Switch/1 -> Multiport Switch/9
  Constant5/1 -> Multiport Switch/4
  Constant2/1 -> Multiport Switch/2
  Constant7/1 -> Multiport Switch/6
  Constant4/1 -> Switch/1
  Constant3/1 -> Multiport Switch/3
  MATLAB Function/1(engine_rpm) -> Chart/1(engine_rpm)
  engine_rpm/1 -> MATLAB Function/1(rpm_in)
  Switch1/1 -> Data Store Write/1
  headlight_status/1 -> Switch1/2
  Constant15/1 -> Multiport Switch2/2
  Constant16/1 -> Multiport Switch2/3
  Constant17/1 -> Multiport Switch2/4
  Constant19/1 -> Multiport Switch2/5
  Constant20/1 -> Multiport Switch2/6
  Constant21/1 -> Multiport Switch2/7
  Constant18/1 -> Multiport Switch2/8
  Constant22/1 -> Multiport Switch2/10
  Constant23/1 -> Switch2/1
  Constant24/1 -> Switch2/3
  Pulse Generator1/1 -> Switch2/2
  Switch2/1 -> Multiport Switch2/9
  Multiport Switch/1 -> Switch1/3
  Multiport Switch2/1 -> Switch1/1

== stateflow chart bench_test_racecar_shiftlight/gear calc1/Chart ==
  state Neutral
    en, du:
    current_gear = 0;
  state Gear_Out
    state In_First
      en, du:
      current_gear = 1;
    state In_Second
      en, du:
      current_gear = 2;
    state In_Third
      en, du:
      current_gear = 3;
    state In_Fourth
      en, du:
      current_gear = 4;
    state In_Fifth
      en, du:
      current_gear = 5;
    state In_Sixth
      en, du:
      current_gear = 6;
  state Clutch_Out
    en, du:
    current_gear = 0;
  state Clutch_In
    en, du:
    current_gear = 0;
  (default) -> Neutral
  Neutral -> Clutch_Out : [clutch_status == 1]
  Clutch_In -> Neutral [order 8] : after(200,msec)
  Clutch_In -> In_First [order 1] : [in_first]
  In_First -> Clutch_In : [~in_first]
  Clutch_In -> In_Second [order 2] : [in_second]
  In_Second -> Clutch_In : [~in_second]
  Clutch_In -> In_Third [order 3] : [in_third]
  Clutch_Out -> Clutch_In : [clutch_status == 0 ...
      | && vehicle_speed >= 5]
  In_Third -> Clutch_In : [~in_third]
  Clutch_In -> Clutch_Out [order 7] : [clutch_status == 1]
  Clutch_In -> In_Fourth [order 4] : [in_forth]
  In_Fourth -> Clutch_In : [~in_forth]
  Clutch_In -> In_Fifth [order 5] : [in_fifth]
  In_Fifth -> Clutch_In : [~in_fifth]
  Clutch_In -> In_Sixth [order 6] : [in_sixth]
  In_Sixth -> Clutch_In : [~in_sixth]
  Gear_Out -> Clutch_Out : [clutch_status == 1]
  data: in_second input; in_first input; in_third input; in_forth input; in_fifth input; in_sixth input; vehicle_speed input; clutch_status input; current_gear output

== stateflow chart bench_test_racecar_shiftlight/gear calc2/Chart ==
  state Start_Up
    en, du:
    current_gear = 8;
  state Neutral
    en, du:
    current_gear = 0;
  state Gear_Out
    state In_First
      en, du:
      current_gear = 1;
    state In_Second
      en, du:
      current_gear = 2;
    state In_Third
      en, du:
      current_gear = 3;
    state In_Fourth
      en, du:
      current_gear = 4;
    state In_Fifth
      en, du:
      current_gear = 5;
    state In_Sixth
      en, du:
      current_gear = 6;
  state Clutch_Out
    en, du:
    current_gear = 0;
  state Clutch_In
    en, du:
    current_gear = 0;
  (default) -> Start_Up
  Start_Up -> Neutral : after(3000,msec)
  Neutral -> Clutch_Out : [clutch_status == 1]
  Clutch_In -> Neutral [order 8] : after(200,msec)
  Clutch_In -> In_First [order 1] : [in_first]
  In_First -> Clutch_In : [~in_first]
  Clutch_In -> In_Second [order 2] : [in_second]
  In_Second -> Clutch_In : [~in_second]
  Clutch_In -> In_Third [order 3] : [in_third]
  Clutch_Out -> Clutch_In : [clutch_status == 0 ...
      | && vehicle_speed >= 5]
  In_Third -> Clutch_In : [~in_third]
  Clutch_In -> Clutch_Out [order 7] : [clutch_status == 1]
  Clutch_In -> In_Fourth [order 4] : [in_forth]
  In_Fourth -> Clutch_In : [~in_forth]
  Clutch_In -> In_Fifth [order 5] : [in_fifth]
  In_Fifth -> Clutch_In : [~in_fifth]
  Clutch_In -> In_Sixth [order 6] : [in_sixth]
  In_Sixth -> Clutch_In : [~in_sixth]
  Gear_Out -> Clutch_Out : [clutch_status == 1]
  data: in_second input; in_first input; in_third input; in_forth input; in_fifth input; in_sixth input; vehicle_speed input; clutch_status input; current_gear output

== stateflow chart bench_test_racecar_shiftlight/gear calc2/clutch_debounce ==
  state Wait
    state To_on
      en, du:
      clutch_debounced = 0;
    state To_off
      en, du:
      clutch_debounced = 1;
  state Off
    en, du:
    clutch_debounced = 0;
  state On
    en, du:
    clutch_debounced = 1;
  (default) -> Off
  Off -> To_on : [clutch_status == 1]
  To_on -> On [order 2] : after(200,msec)
  To_on -> Off [order 1] : [clutch_status == 0]
  To_off -> Off [order 2] : after(200,msec)
  On -> To_off : [clutch_status == 0]
  To_off -> On [order 1] : [clutch_status == 1]
  data: clutch_status input; clutch_debounced output

== stateflow chart bench_test_racecar_shiftlight/Subsystem/Chart ==
  note: Outputs are active low
  state No_Gear
    en, du:
    D0_IN = 0;
    D1_IN = 0;
    D2_IN = 0;
    D3_IN = 0;
  state First_Gear
    en, du:
    D0_IN = 0;
    D1_IN = 1;
    D2_IN = 1;
    D3_IN = 1;
  state Second_Gear
    en, du:
    D0_IN = 1;
    D1_IN = 0;
    D2_IN = 1;
    D3_IN = 1;
  state Third_Gear
    en, du:
    D0_IN = 0;
    D1_IN = 0;
    D2_IN = 1;
    D3_IN = 1;
  state Forth_Gear
    en, du:
    D0_IN = 1;
    D1_IN = 1;
    D2_IN = 0;
    D3_IN = 1;
  state Fifth_Gear
    en, du:
    D0_IN = 0;
    D1_IN = 1;
    D2_IN = 0;
    D3_IN = 1;
  state Sixth_Gear
    en, du:
    D0_IN = 1;
    D1_IN = 0;
    D2_IN = 0;
    D3_IN = 1;
  state Start_Up_Check
    en, du:
    D0_IN = 1;
    D1_IN = 1;
    D2_IN = 1;
    D3_IN = 0;
  (default) -> No_Gear
  No_Gear -> First_Gear [order 1] : [current_gear == 1]
  First_Gear -> No_Gear : [current_gear ~= 1]
  No_Gear -> Second_Gear [order 2] : [current_gear == 2]
  Second_Gear -> No_Gear : [current_gear ~= 2]
  No_Gear -> Third_Gear [order 3] : [current_gear == 3]
  Third_Gear -> No_Gear : [current_gear ~= 3]
  No_Gear -> Forth_Gear [order 4] : [current_gear == 4]
  Forth_Gear -> No_Gear : [current_gear ~= 4]
  No_Gear -> Fifth_Gear [order 5] : [current_gear == 5]
  Fifth_Gear -> No_Gear : [current_gear ~= 5]
  No_Gear -> Sixth_Gear [order 6] : [current_gear == 6]
  Sixth_Gear -> No_Gear : [current_gear ~= 6]
  No_Gear -> Start_Up_Check [order 7] : [current_gear == 8]
  Start_Up_Check -> No_Gear : [current_gear ~= 8]
  data: current_gear input; D0_IN output; D1_IN output; D2_IN output; D3_IN output

== matlab function bench_test_racecar_shiftlight/shiftlight control/MATLAB Function ==
  data: rpm_in input; engine_rpm output
function engine_rpm = startup_ramp(rpm_in)
%#codegen

% ===== Tunable constants =====
Ts = single(0.001);        % MUST match model fixed-step size
rpm_low  = single(5200);
rpm_high = single(6750);

T_up   = single(1.0);
T_hold = single(1.0);
T_down = single(1.0);

T_total = T_up + T_hold + T_down;

slope = (rpm_high - rpm_low) / T_up;   % 1600 rpm/s

% ===== Persistent time counter =====
persistent t
if isempty(t)
    t = single(0.0);
end

% Saturating time accumulator
if t < T_total
    t = t + Ts;
    if t > T_total
        t = T_total;
    end
end

% ===== Piecewise profile =====
if t <= T_up
    % Ramp up (0–1s)
    engine_rpm = rpm_low + slope * t;

elseif t <= (T_up + T_hold)
    % Hold at 6800 (1–3s)
    engine_rpm = rpm_high;

elseif t < T_total
    % Ramp down (3–4s)
    engine_rpm = rpm_high - slope * (t - T_up - T_hold);

else
    % After startup profile → follow input
    engine_rpm = single(rpm_in);
end

== stateflow chart bench_test_racecar_shiftlight/gear calc/Chart ==
  state Init
    en, du:
    current_gear = 0;
  state Idle
    en, du:
    current_gear = 0;
  (default) -> Init
  Idle -> Init
  Init -> Idle
  data: in_second input; in_first input; in_third input; in_forth input; in_fifth input; in_sixth input; vehicle_speed input; current_gear output; clutch_status input

== stateflow chart bench_test_racecar_shiftlight/gear calc1/clutch_debounce ==
  state Wait
    state To_on
      en, du:
      clutch_debounced = 0;
    state To_off
      en, du:
      clutch_debounced = 1;
  state Off
    en, du:
    clutch_debounced = 0;
  state On
    en, du:
    clutch_debounced = 1;
  (default) -> Off
  Off -> To_on : [clutch_status == 1]
  To_on -> On [order 2] : after(200,msec)
  To_on -> Off [order 1] : [clutch_status == 0]
  To_off -> Off [order 2] : after(200,msec)
  On -> To_off : [clutch_status == 0]
  To_off -> On [order 1] : [clutch_status == 1]
  data: clutch_status input; clutch_debounced output

== stateflow chart bench_test_racecar_shiftlight/shiftlight control/Chart ==
  state Init
    en, du:
    shiftlight_stage = 0;
  state stage1
    en, du:
    shiftlight_stage = 1;
  state stage2
    en, du:
    shiftlight_stage = 2;
  state stage3
    en, du:
    shiftlight_stage = 3;
  state stage4
    en, du:
    shiftlight_stage = 4;
  state stage5
    en, du:
    shiftlight_stage = 5;
  state stage6
    en, du:
    shiftlight_stage = 6;
  state stage7
    en, du:
    shiftlight_stage = 7;
  state stage8
    en, du:
    shiftlight_stage = 8;
  (default) -> Init
  Init -> stage1 : [engine_rpm >= 5400]
  stage1 -> Init [order 2] : [engine_rpm < 5400]
  stage1 -> stage2 [order 1] : [engine_rpm >= 5600]
  stage2 -> stage1 [order 1] : [engine_rpm < 5600]
  stage2 -> stage3 [order 2] : [engine_rpm >= 5800]
  stage3 -> stage2 [order 1] : [engine_rpm < 5800]
  stage3 -> stage4 [order 2] : [engine_rpm >= 6000]
  stage4 -> stage3 [order 1] : [engine_rpm < 6000]
  stage4 -> stage5 [order 2] : [engine_rpm >= 6200]
  stage5 -> stage4 [order 1] : [engine_rpm < 6200]
  stage5 -> stage6 [order 2] : [engine_rpm >= 6400]
  stage6 -> stage5 [order 1] : [engine_rpm < 6400]
  stage6 -> stage7 [order 2] : [engine_rpm >= 6600]
  stage7 -> stage6 [order 1] : [engine_rpm < 6600]
  stage7 -> stage8 [order 2] : [engine_rpm >= 6800]
  stage8 -> stage7 : [engine_rpm < 6800]
  data: engine_rpm input; shiftlight_stage output
